simulink model "Copy_2_of_SIMSCAPE_SIM_PROTOTYPE"  (R2025b)
settings: Solver=ode15s  StartTime=0.0  StopTime=T_sim  MaxStep=1e-6  RelTol=1e-6
InitFcn:
  | run param_file_original.m
  | % param = struct();
  | %
  | % % Pressure Rails
  | % param.P_T = 101325;
  | % param.P_H = 7e6;
  | % param.P_M = 3.5e6;
  | % param.P_L = param.P_T;
  | %
  | % % Linear Actuator Chamber
  | % param.V1_0 = 250e-6;
  | % param.Acap = pi*(2.54)^2*1e-4;
  | %
  | % % Intermediary volumes
  | % param.V3_0 = 10e-6;
  | % param.V4_0 = 10e-6;
  | %
  | % % Fluid
  | % param.beta = 1.8e9;
  | % param.air = 0;
  | % param.rho = 870;
  | %
  | % % Valve
  | % param.max_Avt = 4.9160e-06;
  | % param.Cd = 0.6;
  | % param.stroke = 5e-3;
  | %
  | % % Valve Dynamics
  | % param.wn = 50*2*pi;
  | % param.zeta = 1;
  | %
  | % % Hydraulic Pump/Motor
  | % param.J_hyd = 3000e-7;
  | % param.D = 0.8e-6;    % In cc/rev
  | % param.pump_mech_eff = 100*(1/100);
  | % param.pump_vol_eff = 100*(1/100);
  | %
  | % % Electric Motor/Generator
  | % param.J_elec = 3060e-7;
  | % param.Kt = 109e-3;
  | % param.Kv = (88*pi)/30; % In rads^-1/Volt
  | % param.elec_eff = 100*(1/100);
  | % param.max_mech_power = 90;
  | %
  | % % Initial speed
  | % param.start_final_velocity = 100;
values from neighbouring files (symbols this model uses):
  param = struct()    [Copy_of_param_file.m]    (also in param_file.m; param_file_loss_vs_freq.m; param_file_original.m; param_file_turbine.m)
libraries: fl_lib x24, nesl_utility x14, SimscapeFluids_lib x2
settings Model: Creator=user  LastModifiedBy=user
settings SolverCC: MaxConsecutiveMinStep=2  ZeroCrossAlgorithm=Adaptive
settings DebuggingCC: AlgebraicLoopMsg=none

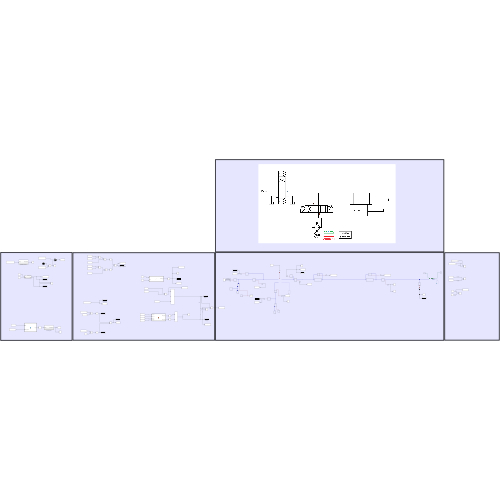
[thumbnail: Simulink's stored preview of the top-level diagram]
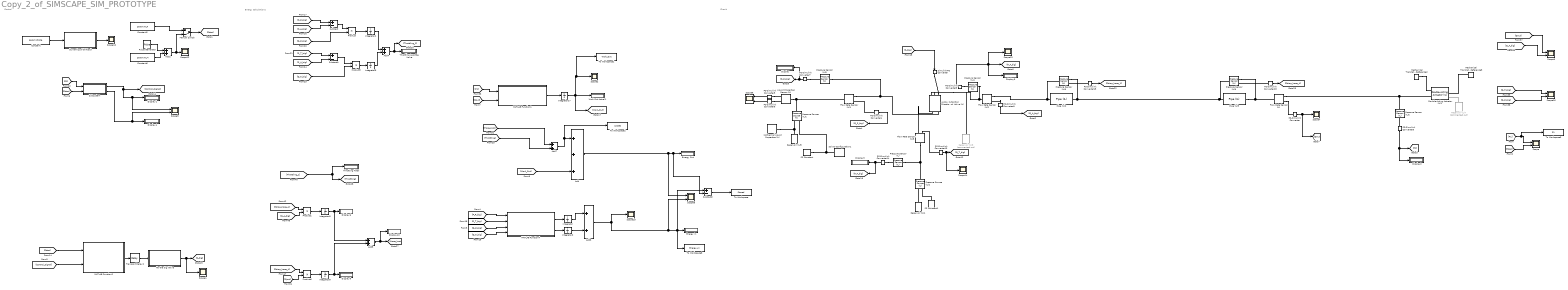
== system Copy_2_of_SIMSCAPE_SIM_PROTOTYPE ==
  note: Control
  note: Energy Calculations
  note: Circuit
  4-Way 2-Position Directional Valve (IL) : SimscapeFluids_lib/Isothermal Liquid/Valves & Orifices/Directional Control Valves/4-Way 2-Position Directional Valve (IL)  open_orifices_pos=fluids.isothermal_liquid.valves_orifices.directional_control_valves.enum.OpenOrifices4Way2Position.PA_BT  open_orifices_neg=fluids.isothermal_liquid.valves_orifices.directional_control_valves.enum.OpenOrifices4Way2Position.PB_AT  area_spec=fluids.isothermal_liquid.valves_orifices.directional_control_valves.enum.directional_valve_area_spec.identical  valve_spec=fluids.isothermal_liquid.valves_orifices.directional_control_valves.enum.directional_valve_spec.linear  del_S_max=param.stroke m  area_max=param.max_Avt m^2  del_S_TLU=[0, .00125, .0025, .00375, .005] m  valve_area_TLU=[1e-10, 1e-05, 4e-05, 6e-05, .0001] m^2  del_S_vol_flow_TLU=[0, .00125, .0025, .00375, .005] m  p_diff_TLU=[-.1, .3, .5, .7] MPa  vol_flow_TLU=[-1e-08, 2.2e-08, 2.8e-08, 3.4e-08; -9e-06, .00015, .0002, .00024; -.00036, .00063, .00081, .00096; -.00054, .00094, .0012, .0014; -.00091, .0016, .002, .0024] m^3/s  p_diff_TLU_const=[-.1, .3, .5, .7] MPa  vol_flow_TLU_const=[-.0009, .0016, .002, .0024] m^3/s  area_const=1e-4 m^2  area_leak=1e-10 m^2  area=inf m^2  Cd=0.64  Re_c=150  smoothing_factor=0.01  pressure_recovery=false  S_max_PA=5e-3 m  del_S_max_PA=0.005 m  area_max_PA=1e-4 m^2  del_S_TLU_PA=[0, .00125, .0025, .00375, .005] m  valve_area_TLU_PA=[1e-10, 1e-05, 4e-05, 6e-05, .0001] m^2  del_S_vol_flow_TLU_PA=[0, .00125, .0025, .00375, .005] m  p_diff_TLU_PA=[-.1, .3, .5, .7] MPa  vol_flow_TLU_PA=[-1e-08, 2.2e-08, 2.8e-08, 3.4e-08; -9e-06, .00015, .0002, .00024; -.00036, .00063, .00081, .00096; -.00054, .00094, .0012, .0014; -.00091, .0016, .002, .0024] m^3/s  area_const_PA=1e-4 m^2  p_diff_TLU_const_PA=[-.1, .3, .5, .7] MPa  vol_flow_TLU_const_PA=[-.0009, .0016, .002, .0024] m^3/s  S_max_PB=-5e-3 m  del_S_max_PB=0.005 m  area_max_PB=1e-4 m^2  del_S_TLU_PB=[0, .00125, .0025, .00375, .005] m  valve_area_TLU_PB=[1e-10, 1e-05, 4e-05, 6e-05, .0001] m^2  del_S_vol_flow_TLU_PB=[0, .00125, .0025, .00375, .005] m  p_diff_TLU_PB=[-.1, .3, .5, .7] MPa  vol_flow_TLU_PB=[-1e-08, 2.2e-08, 2.8e-08, 3.4e-08; -9e-06, .00015, .0002, .00024; -.00036, .00063, .00081, .00096; -.00054, .00094, .0012, .0014; -.00091, .0016, .002, .0024] m^3/s  area_const_PB=1e-4 m^2  p_diff_TLU_const_PB=[-.1, .3, .5, .7] MPa  vol_flow_TLU_const_PB=[-.0009, .0016, .002, .0024] m^3/s  S_max_AT=-5e-3 m  del_S_max_AT=0.005 m  area_max_AT=1e-4 m^2  del_S_TLU_AT=[0, .00125, .0025, .00375, .005] m  valve_area_TLU_AT=[1e-10, 1e-05, 4e-05, 6e-05, .0001] m^2  del_S_vol_flow_TLU_AT=[0, .00125, .0025, .00375, .005] m  p_diff_TLU_AT=[-.1, .3, .5, .7] MPa  vol_flow_TLU_AT=[-1e-08, 2.2e-08, 2.8e-08, 3.4e-08; -9e-06, .00015, .0002, .00024; -.00036, .00063, .00081, .00096; -.00054, .00094, .0012, .0014; -.00091, .0016, .002, .0024] m^3/s  area_const_AT=1e-4 m^2  p_diff_TLU_const_AT=[-.1, .3, .5, .7] MPa  vol_flow_TLU_const_AT=[-.0009, .0016, .002, .0024] m^3/s  S_max_BT=5e-3 m  del_S_max_BT=0.005 m  area_max_BT=1e-4 m^2  del_S_TLU_BT=[0, .00125, .0025, .00375, .005] m  valve_area_TLU_BT=[1e-10, 1e-05, 4e-05, 6e-05, .0001] m^2  del_S_vol_flow_TLU_BT=[0, .00125, .0025, .00375, .005] m  p_diff_TLU_BT=[-.1, .3, .5, .7] MPa  vol_flow_TLU_BT=[-1e-08, 2.2e-08, 2.8e-08, 3.4e-08; -9e-06, .00015, .0002, .00024; -.00036, .00063, .00081, .00096; -.00054, .00094, .0012, .0014; -.00091, .0016, .002, .0024] m^3/s  area_const_BT=1e-4 m^2  p_diff_TLU_const_BT=[-.1, .3, .5, .7] MPa  vol_flow_TLU_const_BT=[-.0009, .0016, .002, .0024] m^3/s
      settings: InternalSimscapePortConfiguration="{\"Bottom\":[{\"id\":\"P\",\"label\":\"P\",\"type\":\"foundation.isothermal_liquid.isothermal_liquid\"},{\"id\":\"T\",\"label\":\"T\",\"type\":\"foundation.isothermal_liquid.isothermal_liquid\"}],\"Left\":[{\"id\":\"S\",\"label\":\"S\",\"type\":\"input\"}],\"Right\":[],\"Top\":[{\"id\":\"A\",\"label\":\"A\",\"type\":\"foundation.isothermal_liquid.isothermal_liquid\"},{\"id\":\"B\",\"label\":\"B\",\"type\":\"foundation.isothermal_liquid.isothermal_liquid\"}]}"
  Add : Sum  Inputs=+++
  Add{2..5,7} (5 alike) : Sum
  Constant : Constant  Value=param.stroke
  Constant2 : Constant  Value=param.P_H
  Constant6 : Constant  Value=param.P_M
  Display{,1..6,9..10} (9 alike) : Display
  Double-Acting Actuator (IL)1 : SimscapeFluids_lib/Isothermal Liquid/Actuators/Double-Acting Actuator (IL)  single_fluid=true  mech_orientation=foundation.enum.MechOrientationTranslational.Positive  piston_area_A=param.Acap m^2  piston_area_B=4e-4 m^2  stroke=param.V1_0/param.Acap m  dead_volume_A=1e-5 m^3  dead_volume_B=1e-5 m^3  pressure_spec=foundation.enum.pressure_spec.atmospheric  environment_pressure=0.101325 MPa  hardstop_model=simscape.enum.hardstop.smooth  stiff_coeff=1e10 N/m  damping_coeff=150 N*s/m  transition=0.1 mm  coeff_rest=0.7  v_tol=0.001 m/s  f_tol=0.001 N  cushion_A_spec=false  area_plunger_A=1e-4 m^2  length_plunger_A=1e-3 m  area_cushion_orifice_A=1e-6 m^2  area_leak_plunger_A=1e-7 m^2  p_crack_differential_A=0.01 MPa  press_max_differential_A=0.1 MPa  check_valve_area_max_A=1e-4 m^2  check_valve_area_leak_A=1e-10 m^2  smoothing_factor_A=0.01  cushion_B_spec=false  area_plunger_B=1e-4 m^2  length_plunger_B=1e-3 m  area_cushion_orifice_B=1e-6 m^2  area_leak_plunger_B=1e-7 m^2  p_crack_differential_B=0.01 MPa  press_max_differential_B=0.1 MPa  check_valve_area_max_B=1e-4 m^2  check_valve_area_leak_B=1e-10 m^2  smoothing_factor_B=0.01  friction_spec=false  breakaway_Coulomb_ratio=1.2  breakaway_velocity=0.1 m/s  preload_force=20 N  Coulomb_coeff=1e-6 N/Pa  viscous_coeff=100 N*s/m  leakage_spec=false  clearance=1e-4 m  piston_length=0.01 m  displacement_spec=foundation.enum.DisplacementSpec.Calculate  x0=param.V1_0/param.Acap m  dynamic_compressibility=true  p0_A=param.P_initial + param.P_T Pa  p0_B=param.P_T Pa  p_nominal_A=0.101325 MPa  p_nominal_B=0.101325 MPa
      settings: InternalSimscapePortConfiguration="{\"Bottom\":[],\"Left\":[{\"id\":\"C\",\"label\":\"C\",\"type\":\"foundation.mechanical.translational.translational\"},{\"id\":\"A\",\"label\":\"A\",\"type\":\"foundation.isothermal_liquid.isothermal_liquid\"}],\"Right\":[{\"id\":\"p_out\",\"label\":\"p\",\"type\":\"output\"},{\"id\":\"R\",\"label\":\"R\",\"type\":\"foundation.mechanical.translational.translational\"},{\"id\":\"B\",\"label\":\"B\",\"type\":\"foundation.isothermal_liquid.isothermal_liquid\"}],\"Top\":[]}"
  Dynamics of Orifice 3 : Subsystem
  Energy In : Display
  Energy Out : Display
  Flow Rate Sensor (IL){,1..2,5} (4 alike) : fl_lib/Isothermal Liquid/Sensors/Flow Rate Sensor (IL)  sensor_type=foundation.enum.mass_volumetric_sensor.volumetric
      settings: InternalSimscapePortConfiguration="{\"Bottom\":[],\"Left\":[{\"id\":\"A\",\"label\":\"A\",\"type\":\"foundation.isothermal_liquid.isothermal_liquid\"}],\"Right\":[{\"id\":\"B\",\"label\":\"B\",\"type\":\"foundation.isothermal_liquid.isothermal_liquid\"},{\"id\":\"V\",\"label\":\"V\",\"type\":\"output\"}],\"Top\":[]}"
  For the big Valve : Subsystem
  Integrator{,1..3,5,9,17} (7 alike) : Integrator
  Isothermal Liquid Properties (IL) : fl_lib/Isothermal Liquid/Utilities/Isothermal Liquid Properties (IL)  rho_L_atm=param.rho kg/m^3  bulk_modulus_model=foundation.enum.bulk_modulus_model.const  beta_gain=6  beta_L_atm=param.beta Pa  nu_atm=1.0034e-6 m^2/s  p_atm=0.101325 MPa  p_min=1 Pa  properties_range_check=simscape.enum.assert.action.error  air_fraction=0.005  polytropic_index=1.0  rho_g_atm=1.225 kg/m^3  air_dissolution_model=false  p_crit=1 MPa
  Liquid Properties Sensor (IL) : fl_lib/Isothermal Liquid/Sensors/Liquid Properties Sensor (IL)  density_measure=false  bulk_modulus_measure=true  entrained_air_measure=true
      settings: InternalSimscapePortConfiguration="{\"Bottom\":[],\"Left\":[{\"id\":\"A\",\"label\":\"A\",\"type\":\"foundation.isothermal_liquid.isothermal_liquid\"}],\"Right\":[{\"id\":\"beta\",\"label\":\"beta\",\"type\":\"output\"},{\"id\":\"theta\",\"label\":\"theta\",\"type\":\"output\"}],\"Top\":[]}"
  MATLAB Function1 : MATLAB Function  TreatAsAtomicUnit=on
  MATLAB Function2 : MATLAB Function  TreatAsAtomicUnit=on
  MATLAB Function4 : MATLAB Function  TreatAsAtomicUnit=on
  Manual Switch : ManualSwitch  CurrentSetting=0
  Mechanical Translational Reference2 : fl_lib/Mechanical/Translational Elements/Mechanical Translational Reference
  Mechanical Translational Reference3 : fl_lib/Mechanical/Translational Elements/Mechanical Translational Reference
  PS Constant : fl_lib/Physical Signals/Sources/PS Constant  constant=param.P_H Pa
  PS Constant1 : fl_lib/Physical Signals/Sources/PS Constant  constant=param.P_M Pa
  PS-Simulink Converter : nesl_utility/PS-Simulink Converter  PhysicalDomain=network_engine_domain  SubClassName=ps_output  LeftPortType=input  RightPortType=output  PseudoPeriodic=off  Frequencies=[]  VectorFormat=inherit  Unit=m^3/s  AffineConversion=off
  PS-Simulink Converter{3..9,13..15,18} (11 alike) : nesl_utility/PS-Simulink Converter  PhysicalDomain=network_engine_domain  SubClassName=ps_output  LeftPortType=input  RightPortType=output  PseudoPeriodic=off  Frequencies=[]  VectorFormat=inherit  Unit=inherit  AffineConversion=off
  Pipe (IL)2 : fl_lib/Isothermal Liquid/Elements/Pipe (IL)  length=0.2 m  area=0.25*pi*(param.D_hose)^2 mm^2  Dh=param.D_hose mm  length_add=0.5 m  roughness=15e-6 m  Re_lam=2000  Re_tur=4000  shape_factor=64  dynamic_compressibility=true  inertia=false  p0=param.P_initial+param.P_T Pa  mdot0=0 kg/s
      settings: InternalSimscapePortConfiguration="{\"Bottom\":[],\"Left\":[{\"id\":\"A\",\"label\":\"A\",\"type\":\"foundation.isothermal_liquid.isothermal_liquid\"}],\"Right\":[{\"id\":\"B\",\"label\":\"B\",\"type\":\"foundation.isothermal_liquid.isothermal_liquid\"}],\"Top\":[]}"
  Pipe (IL)5 : fl_lib/Isothermal Liquid/Elements/Pipe (IL)  length=1 m  area=0.25*pi*(param.D_hose)^2 mm^2  Dh=param.D_hose mm  length_add=0.5 m  roughness=15e-6 m  Re_lam=2000  Re_tur=4000  shape_factor=64  dynamic_compressibility=true  inertia=false  p0=param.P_initial+param.P_T Pa  mdot0=0 kg/s
      settings: InternalSimscapePortConfiguration="{\"Bottom\":[],\"Left\":[{\"id\":\"A\",\"label\":\"A\",\"type\":\"foundation.isothermal_liquid.isothermal_liquid\"}],\"Right\":[{\"id\":\"B\",\"label\":\"B\",\"type\":\"foundation.isothermal_liquid.isothermal_liquid\"}],\"Top\":[]}"
  Pressure Sensor (IL){,2..4} (4 alike) : fl_lib/Isothermal Liquid/Sensors/Pressure Sensor (IL)  pressure_measure=foundation.enum.pressure_measure.gauge
      settings: InternalSimscapePortConfiguration="{\"Bottom\":[],\"Left\":[{\"id\":\"A\",\"label\":\"A\",\"type\":\"foundation.isothermal_liquid.isothermal_liquid\"}],\"Right\":[{\"id\":\"Pg\",\"label\":\"Pg\",\"type\":\"output\"}],\"Top\":[]}"
  Pressure Sensor (IL)6 : fl_lib/Isothermal Liquid/Sensors/Pressure Sensor (IL)  pressure_measure=foundation.enum.pressure_measure.difference
      settings: InternalSimscapePortConfiguration="{\"Bottom\":[],\"Left\":[{\"id\":\"A\",\"label\":\"A\",\"type\":\"foundation.isothermal_liquid.isothermal_liquid\"}],\"Right\":[{\"id\":\"B\",\"label\":\"B\",\"type\":\"foundation.isothermal_liquid.isothermal_liquid\"},{\"id\":\"P\",\"label\":\"P\",\"type\":\"output\"}],\"Top\":[]}"
  Pressure Sensor (IL)9 : fl_lib/Isothermal Liquid/Sensors/Pressure Sensor (IL)  pressure_measure=foundation.enum.pressure_measure.difference
      settings: InternalSimscapePortConfiguration="{\"Bottom\":[],\"Left\":[{\"id\":\"A\",\"label\":\"A\",\"type\":\"foundation.isothermal_liquid.isothermal_liquid\"}],\"Right\":[{\"id\":\"B\",\"label\":\"B\",\"type\":\"foundation.isothermal_liquid.isothermal_liquid\"},{\"id\":\"P\",\"label\":\"P\",\"type\":\"output\"}],\"Top\":[]}"
  Pressure Source (IL)1 : fl_lib/Isothermal Liquid/Sources/Pressure Source (IL)  source_type=foundation.enum.constant_controlled.controlled  pressure_differential=0 MPa
      settings: InternalSimscapePortConfiguration="{\"Bottom\":[],\"Left\":[{\"id\":\"A\",\"label\":\"A\",\"type\":\"foundation.isothermal_liquid.isothermal_liquid\"},{\"id\":\"P\",\"label\":\"P\",\"type\":\"input\"}],\"Right\":[{\"id\":\"B\",\"label\":\"B\",\"type\":\"foundation.isothermal_liquid.isothermal_liquid\"}],\"Top\":[]}"
  Pressure Source (IL)2 : fl_lib/Isothermal Liquid/Sources/Pressure Source (IL)  source_type=foundation.enum.constant_controlled.controlled  pressure_differential=0 MPa
      settings: InternalSimscapePortConfiguration="{\"Bottom\":[],\"Left\":[{\"id\":\"A\",\"label\":\"A\",\"type\":\"foundation.isothermal_liquid.isothermal_liquid\"},{\"id\":\"P\",\"label\":\"P\",\"type\":\"input\"}],\"Right\":[{\"id\":\"B\",\"label\":\"B\",\"type\":\"foundation.isothermal_liquid.isothermal_liquid\"}],\"Top\":[]}"
  Product{,1,3,6} (4 alike) : Product
  Pulse Generator : DiscretePulseGenerator  PulseType=Time based  Amplitude=param.P_H-param.P_M  Period=param.T_period  PulseWidth=50  PhaseDelay=param.delay
  Reservoir (IL)1 : fl_lib/Isothermal Liquid/Elements/Reservoir (IL)  reservoir_type=foundation.enum.constant_controlled.constant  pressure_spec=foundation.enum.pressure_spec.atmospheric  reservoir_pressure=0.101325 MPa
  Reservoir (IL)5 : fl_lib/Isothermal Liquid/Elements/Reservoir (IL)  reservoir_type=foundation.enum.constant_controlled.constant  pressure_spec=foundation.enum.pressure_spec.atmospheric  reservoir_pressure=0.101325 MPa
  Reservoir (IL)7 : fl_lib/Isothermal Liquid/Elements/Reservoir (IL)  Commented=on  reservoir_type=foundation.enum.constant_controlled.constant  pressure_spec=foundation.enum.pressure_spec.atmospheric  reservoir_pressure=0.101325 MPa
  Reservoir (IL)8 : fl_lib/Isothermal Liquid/Elements/Reservoir (IL)  Commented=on  reservoir_type=foundation.enum.constant_controlled.constant  pressure_spec=foundation.enum.pressure_spec.atmospheric  reservoir_pressure=0.101325 MPa
  Scope{,5..6,8..9,16} (6 alike) : Scope  NumInputPorts=2
      Scope settings: ActiveDisplayYMinimum=2.88105870012E+6  ActiveDisplayYMaximum=8.05722169896E+6
      Scope16 settings: ActiveDisplayYMinimum=-0.0002  ActiveDisplayYMaximum=0.00036  DataLoggingVariableName=ScopeData2
      Scope5 settings: ActiveDisplayYMinimum=-0.125  ActiveDisplayYMaximum=1.125  DataLoggingVariableName=ScopeData5
      Scope6 settings: ActiveDisplayYMinimum=0.9  ActiveDisplayYMaximum=1.1  DataLoggingVariableName=ScopeData2
      Scope8 settings: ActiveDisplayYMinimum=-0.5259  ActiveDisplayYMaximum=4.73307
      Scope9 settings: ActiveDisplayYMinimum=-0.0002  ActiveDisplayYMaximum=0.00036
  Scope{1..2,7,10,12..15} (8 alike) : Scope
      Scope1 settings: ActiveDisplayYMinimum=-0.00625  ActiveDisplayYMaximum=0.00625  DataLoggingVariableName=ScopeData3
      Scope10 settings: ActiveDisplayYMinimum=-0.00062  ActiveDisplayYMaximum=0.00562  DataLoggingVariableName=ScopeData3
      Scope12 settings: ActiveDisplayYMinimum=6.0E+6  ActiveDisplayYMaximum=8.0E+6
      Scope13 settings: ActiveDisplayYMinimum=-953073.24084  ActiveDisplayYMaximum=8.17987904394E+6  DataLoggingVariableName=ScopeData7
      Scope14 settings: ActiveDisplayYMinimum=-0.00017  ActiveDisplayYMaximum=0.00017  DataLoggingVariableName=ScopeData8
      Scope2 settings: ActiveDisplayYMinimum=-0.3371  ActiveDisplayYMaximum=3.02982
      Scope7 settings: ActiveDisplayYMinimum=-0.00018  ActiveDisplayYMaximum=0.00017
  Simulink-PS Converter : nesl_utility/Simulink-PS Converter  PhysicalDomain=network_engine_domain  SubClassName=ps_input  LeftPortType=input  RightPortType=output  PseudoPeriodic=off  Frequencies=[]  NoiseDistribution=none  NoiseParameters=[]  Unit=1  AffineConversion=off  FilteringAndDerivatives=provide  SimscapeFilterOrder=1  InputFilterTimeConstant=0.001  UdotUserProvided=0
  Solver Configuration1 : nesl_utility/Solver Configuration  PhysicalDomain=network_engine_domain  SubClassName=solver  LeftPortType=input  RightPortType=generic  Tones=[]  Harmonics=[]  SimulateNoise=off  Profile=off  UseLocalSampling=off  EnableSwitchedLinearOptims=on  FrequencyDomain=off  UseCCode=off  RelTol=0.001  AbsTol=0.001  MinStep=1e-09  ToWorkspace=off  RevertToSquareIcSolve=off  NumHomotopyIterations=100  PhasorMode=off  PhasorModeNumHarmonics=1  ConsistencySolver=NEWTON_XTOL_AFTER_FTOL  IndexReductionMethod=DerivativeReplacement  DoDC=off  ResidualTolerance=1e-09  ConsistencyTolSource=GLOBAL  ConsistencyAbsTol=0.001  ConsistencyRelTol=0.001  ConsistencyTolFactor=0.001  UseLocalSolver=off  LocalSolverChoice=NE_BACKWARD_EULER_ADVANCER  ResolveIndetEquations=on  FunctionEvalNumThread=1  LocalSolverSampleTime=0.001  DoFixedCost=off  MaxNonlinIter=3  MaxModeIter=2  ComputeImpulses=off  ImpulseIterations=2  LinearAlgebra=auto  LinearAlgebraNumThread=0  EquationFormulation=NE_TIME_EF  DelaysMemoryBudget=1024  AutomaticFiltering=on  FilteringTimeConstant=0.001  PartitionStorageMethod=AS_NEEDED  PartitionMemoryBudget=1024  PartitionMethod=ROBUST  MultibodyUseLocalSolver=off  MultibodyLocalSolverChoice=ODE1  MultibodyLocalSolverSampleTime=0.001
  Subsystem : Subsystem
  Subtract : Sum  Inputs=+-
  Subtract1 : Sum  Inputs=+-
  Subtract2 : Sum  Inputs=+-
  Throttling Loss Big Valve : Display
  Throttling Total : Display
  To Workspace : ToWorkspace  VariableName=Stored  SaveFormat=Timeseries  SampleTime=-1
  To Workspace1 : ToWorkspace  VariableName=Work_Out  SaveFormat=Timeseries  SampleTime=-1
  To Workspace2 : ToWorkspace  VariableName=Losses  SaveFormat=Timeseries  SampleTime=-1
  To Workspace3 : ToWorkspace  VariableName=P1  SaveFormat=Timeseries  SampleTime=-1
  To Workspace8 : ToWorkspace  VariableName=Energy_In  SaveFormat=Timeseries  SampleTime=-1
  Transport Delay2 : TransportDelay  DelayTime=param.delay_switch  InitialOutput=param.initial_stroke  BufferSize=1024*105
  Work Out Actual1 : Display
  wires:
  [P1] -> Subsystem/1(P1)
  Subsystem/1(Control_Signal) -> [Control_Signal], Scope5/1, Display1/1
  [Pdes] -> Subsystem/2(Pdes)
  PS-Simulink Converter3/1 -> [P1], Display2/1
  Subsystem/2(delP) -> Scope5/2, Display4/1
  PS-Simulink Converter5/1 -> Scope6/1  "Entrained Air"
  PS-Simulink Converter6/1 -> Scope6/2  "Bulk Modulus"
  PS-Simulink Converter/1 -> [Qout], Scope7/1
  Constant/1 -> Dynamics of Orifice 3/1(Stroke)
  Dynamics of Orifice 3/1(Spool Opening) -> Scope10/1
  PS-Simulink Converter9/1 -> [Q_A_big]
  PS-Simulink Converter4/1 -> [Q_P_big]
  PS-Simulink Converter8/1 -> Display5/1, Scope13/1, [P_A_big]
  [P_P_big] -> MATLAB Function4/1(P_H_rail)
  [Q_P_big] -> MATLAB Function4/3(Q_P_big)
  MATLAB Function1/1(Power_out) -> Integrator17/1
  Integrator17/1 -> To Workspace1/1, Scope2/1, Work Out Actual1/1, [Work_Out]
  [P1] -> MATLAB Function1/1(P1)
  [Qout] -> MATLAB Function1/2(Qout)
  [Work_Out] -> Add/3
  Add/1 -> Subtract2/2, Energy Out/1, Scope8/1  "Out"
  Add3/1 -> Scope8/2, Subtract2/1, To Workspace8/1, Energy In/1, Scope15/1  "In"
  PS-Simulink Converter13/1 -> Scope14/1, [Q_T_big]
  PS-Simulink Converter7/1 -> Display/1, [P_P_big]
  MATLAB Function2/1(S_big) -> Transport Delay2/1
  [Control_Signal] -> MATLAB Function2/2(Control_signal)
  [Pdes] -> MATLAB Function2/1(Pdes)
  [S_big] -> Simulink-PS Converter/1
  For the big Valve/1(Spool Opening) -> Scope1/1, [S_big]
  PS-Simulink Converter14/1 -> [P_T_big], Display3/1
  [P_T_big] -> MATLAB Function4/2(P_M_rail)
  [Q_T_big] -> MATLAB Function4/4(Q_T_big)
  MATLAB Function4/1(Power_out_1) -> Integrator/1
  MATLAB Function4/2(Power_out_2) -> Integrator2/1
  Integrator/1 -> Add3/1
  Integrator2/1 -> Add3/2
  [P_P_big] -> Subtract/1
  [P_A_big] -> Subtract/2
  [Q_P_big] -> Product/2
  Subtract/1 -> Product/1
  Product/1 -> Integrator1/1
  Integrator1/1 -> Add4/1
  Subtract1/1 -> Product3/1
  [Q_T_big] -> Product3/2
  Product3/1 -> Integrator3/1
  Integrator3/1 -> Add4/2
  Add4/1 -> [Throttling_1], Throttling Loss Big Valve/1
  [Throttling] -> Add7/2
  [Qout] -> Scope9/1  "Qout"
  [Q_A_big] -> Scope9/2  "Q_A_big"
  PS-Simulink Converter15/1 -> [Pdrop_hose_1]
  PS-Simulink Converter18/1 -> [Pdrop_hose_4]
  [P_T_big] -> Subtract1/1
  [P_A_big] -> Subtract1/2
  [Q_T_big] -> Scope16/1  "Q_T_big"
  [Q_P_big] -> Scope16/2  "Q_P_big"
  [Pdrop_hose_1] -> Product1/1
  [Q_A_big] -> Product1/2
  Product1/1 -> Integrator5/1
  Integrator5/1 -> Display6/1, Add5/1
  [Pdrop_hose_4] -> Product6/1
  [Qout] -> Product6/2
  Product6/1 -> Integrator9/1
  Integrator9/1 -> Add5/2, Display9/1
  Add5/1 -> Display10/1, [Hose_loss]
  [Throttling_1] -> [Throttling], Throttling Total/1
  [P1] -> To Workspace3/1, Scope/1  "P1"
  [Pdes] -> Scope/2  "Pdes"
  Transport Delay2/1 -> For the big Valve/1(Stroke)
  Subtract2/1 -> To Workspace/1
  Manual Switch/1 -> [Pdes]
  Add2/1 -> Manual Switch/2, Scope12/1
  Pulse Generator/1 -> Add2/1
  Constant2/1 -> Manual Switch/1
  Constant6/1 -> Add2/2
  [Hose_loss] -> Add7/1
  Add7/1 -> To Workspace2/1, Add/1
  connections:
  Solver Configuration1/RConn1 -- PS Constant/RConn1 -- Pressure Source (IL)1/LConn2
  Reservoir (IL)5/LConn1 -- Isothermal Liquid Properties (IL)/RConn1 -- Pressure Source (IL)1/LConn1
  Mechanical Translational Reference2/LConn1 -- Double-Acting Actuator (IL)1/LConn1
  Mechanical Translational Reference3/LConn1 -- Double-Acting Actuator (IL)1/RConn2
  Reservoir (IL)7/LConn1 -- Double-Acting Actuator (IL)1/RConn3
  Flow Rate Sensor (IL)/RConn1 -- Double-Acting Actuator (IL)1/LConn2 -- Pressure Sensor (IL)2/LConn1
  PS-Simulink Converter3/LConn1 -- Pressure Sensor (IL)2/RConn1
  Pressure Sensor (IL)4/LConn1 -- 4-Way 2-Position Directional Valve (IL)/LConn2 -- Flow Rate Sensor (IL)2/LConn1
  PS-Simulink Converter5/LConn1 -- Liquid Properties Sensor (IL)/RConn2
  PS-Simulink Converter6/LConn1 -- Liquid Properties Sensor (IL)/RConn1
  Flow Rate Sensor (IL)/RConn2 -- PS-Simulink Converter/LConn1
  Pipe (IL)5/LConn1 -- Pressure Sensor (IL)9/RConn1 -- Flow Rate Sensor (IL)/LConn1
  Liquid Properties Sensor (IL)/LConn1 -- Pressure Source (IL)1/RConn1 -- Flow Rate Sensor (IL)1/LConn1
  Pressure Sensor (IL)3/LConn1 -- 4-Way 2-Position Directional Valve (IL)/RConn1 -- Flow Rate Sensor (IL)1/RConn1
  Flow Rate Sensor (IL)2/RConn1 -- Pressure Sensor (IL)6/LConn1 -- Pipe (IL)2/LConn1
  PS-Simulink Converter7/LConn1 -- Pressure Sensor (IL)3/RConn1
  PS-Simulink Converter8/LConn1 -- Pressure Sensor (IL)4/RConn1
  PS-Simulink Converter9/LConn1 -- Flow Rate Sensor (IL)2/RConn2
  PS Constant1/RConn1 -- Pressure Source (IL)2/LConn2
  Reservoir (IL)1/LConn1 -- Pressure Source (IL)2/LConn1
  Flow Rate Sensor (IL)5/LConn1 -- Pressure Sensor (IL)/LConn1 -- Pressure Source (IL)2/RConn1
  Flow Rate Sensor (IL)5/RConn1 -- 4-Way 2-Position Directional Valve (IL)/RConn2
  PS-Simulink Converter13/LConn1 -- Flow Rate Sensor (IL)5/RConn2
  PS-Simulink Converter4/LConn1 -- Flow Rate Sensor (IL)1/RConn2
  Pressure Sensor (IL)9/LConn1 -- Pipe (IL)2/RConn1 -- Pressure Sensor (IL)6/RConn1 -- Pipe (IL)5/RConn1
  Simulink-PS Converter/RConn1 -- 4-Way 2-Position Directional Valve (IL)/LConn1
  4-Way 2-Position Directional Valve (IL)/LConn3 -- Reservoir (IL)8/LConn1
  PS-Simulink Converter14/LConn1 -- Pressure Sensor (IL)/RConn1
  PS-Simulink Converter15/LConn1 -- Pressure Sensor (IL)6/RConn2
  PS-Simulink Converter18/LConn1 -- Pressure Sensor (IL)9/RConn2

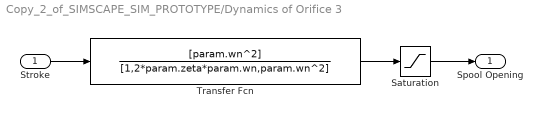
== system Copy_2_of_SIMSCAPE_SIM_PROTOTYPE/Dynamics of Orifice 3 ==
  Stroke : Inport
  Saturation : Saturate  UpperLimit=param.stroke  LowerLimit=0
  Transfer Fcn : TransferFcn  Numerator=[param.wn^2]  Denominator=[1,2*param.zeta*param.wn,param.wn^2]
  Spool Opening : Outport
  wires:
  Transfer Fcn/1 -> Saturation/1
  Saturation/1 -> Spool Opening/1
  Stroke/1 -> Transfer Fcn/1

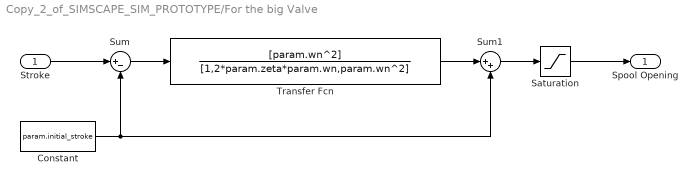
== system Copy_2_of_SIMSCAPE_SIM_PROTOTYPE/For the big Valve ==
  Stroke : Inport
  Constant : Constant  Value=param.initial_stroke
  Saturation : Saturate  UpperLimit=param.stroke  LowerLimit=-param.stroke
  Sum : Sum  Inputs=|+-
  Sum1 : Sum  Inputs=|++
  Transfer Fcn : TransferFcn  Numerator=[param.wn^2]  Denominator=[1,2*param.zeta*param.wn,param.wn^2]
  Spool Opening : Outport
  wires:
  Saturation/1 -> Spool Opening/1
  Sum1/1 -> Saturation/1
  Transfer Fcn/1 -> Sum1/1
  Sum/1 -> Transfer Fcn/1
  Stroke/1 -> Sum/1
  Constant/1 -> Sum1/2, Sum/2

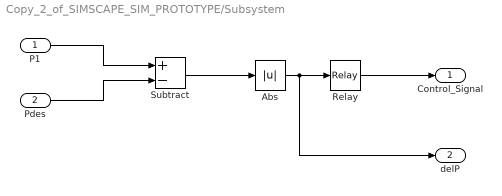
== system Copy_2_of_SIMSCAPE_SIM_PROTOTYPE/Subsystem ==
  P1 : Inport
  Pdes : Inport  Port=2
  Abs : Abs  SaturateOnIntegerOverflow=off
  Relay : Relay  OnSwitchValue=6e5  OffSwitchValue=1e3  OnOutputValue=0  OffOutputValue=1
  Subtract : Sum  Inputs=+-
  Control_Signal : Outport
  delP : Outport  Port=2
  wires:
  P1/1 -> Subtract/1
  Pdes/1 -> Subtract/2
  Subtract/1 -> Abs/1
  Abs/1 -> delP/1, Relay/1
  Relay/1 -> Control_Signal/1

== matlab function Copy_2_of_SIMSCAPE_SIM_PROTOTYPE/MATLAB Function2 ==
  data: Pdes input; S_big output; param parameter; Control_signal input
function S_big  = fcn(Pdes, param, Control_signal)

if Pdes == param.P_H && Control_signal == 0
    S_big = param.stroke;
elseif Pdes == param.P_M && Control_signal == 0
    S_big = -param.stroke;
elseif Pdes == param.P_H && Control_signal > 0
    S_big = param.stroke;
elseif Pdes == param.P_M && Control_signal > 0
    S_big = -param.stroke;
else
    S_big = 0;
end

== matlab function Copy_2_of_SIMSCAPE_SIM_PROTOTYPE/MATLAB Function4 ==
  data: P_H_rail input; P_M_rail input; Q_P_big input; Q_T_big input; Power_out_1 output; Power_out_2 output
function [Power_out_1, Power_out_2] = fcn(P_H_rail, P_M_rail, Q_P_big, Q_T_big)

Power_out_1 = (Q_P_big)*(P_H_rail);

Power_out_2 = (Q_T_big)*(P_M_rail);

== matlab function Copy_2_of_SIMSCAPE_SIM_PROTOTYPE/MATLAB Function1 ==
  data: P1 input; Qout input; Power_out output; param parameter
function Power_out = fcn(P1, Qout, param)

gamma = 1.4; % Adiabatic process
Pt = param.P_T;

Pg = P1-Pt;   % Gauge pressure
r = P1/Pt;    % Pressure ratio
e = exp(Pg/param.beta);
rv = (1/e+param.air*r^(-1/gamma))/(1+param.air);      %Volume ratio

El=param.beta*(e-(1+Pg/param.beta))+Pt*(e-1);           %Energy in liquid
Eg=P1/(gamma-1).*(1-r.^(1/gamma-1));          %Energy in gas
E=(El./e+param.air*Eg.*r.^(-1/gamma))./(1./e+param.air*r.^(-1/gamma));    %Energy in mixture
W = E-(1./rv-1)*Pt;  %Compressibility (volumetric) energy density

Power_out = (Qout)*(W+Pg);
